simulink model "pathFollowingRobotPerturb"  (R2024b)
settings: Solver=VariableStepAuto  StartTime=0.0  StopTime=10000  RelTol=1e-3
undefined symbols (not defined in the file): a, angles, du, dw, dx, dy, initPose, leftPerturbT, mapMaxDimension, maxAngSpeed, maxLinSpeed, minAngSpeed, minLinSpeed, pathpoints, q1, q2, q3, q4, q5, q6, rightPerturbT, sampleTime, speeds
libraries: rllib x1
settings Model: SimulationMode=accelerator  SnapshotBufferSize=100  SnapshotInterval=100  PacingRate=1000  Creator=jose6  LastModifiedBy=jose6
settings DataIOCC: InspectSignalLogs=on

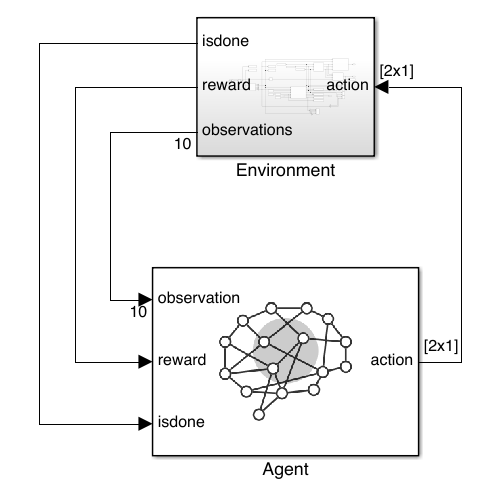
[thumbnail: Simulink's stored preview of the top-level diagram]
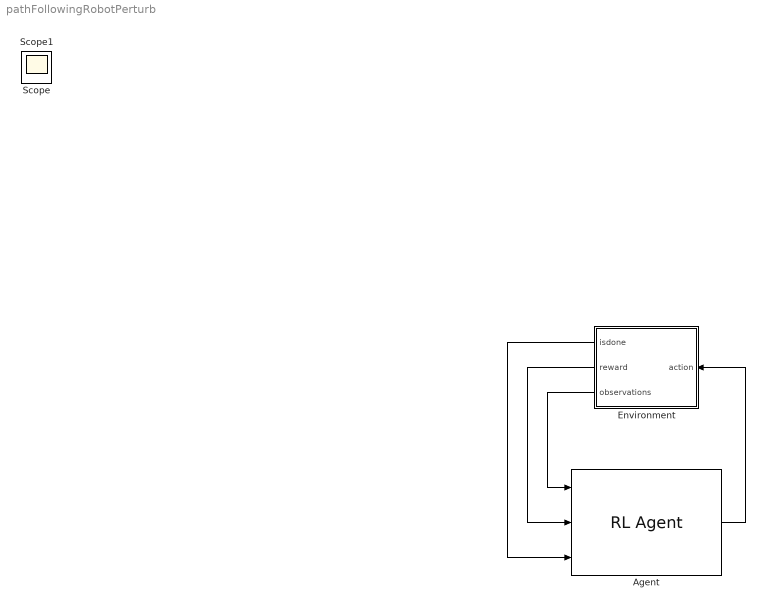
== system pathFollowingRobotPerturb ==
  Agent : rllib/RL Agent  Agent=agent  ExternalActionAsInput=off  ProvideLastAction=off  ProvideCumRwd=off  TreatAsDirectFeedthrough=on  UseStrictObservationDataTypes=off
  Environment : Subsystem
  Scope : Scope
  Scope1 : Scope
  wires:
  Agent/1 -> Environment/1(action)
  Environment/1(isdone) -> Agent/3
  Environment/2(reward) -> Agent/2
  Environment/3(observations) -> Agent/1

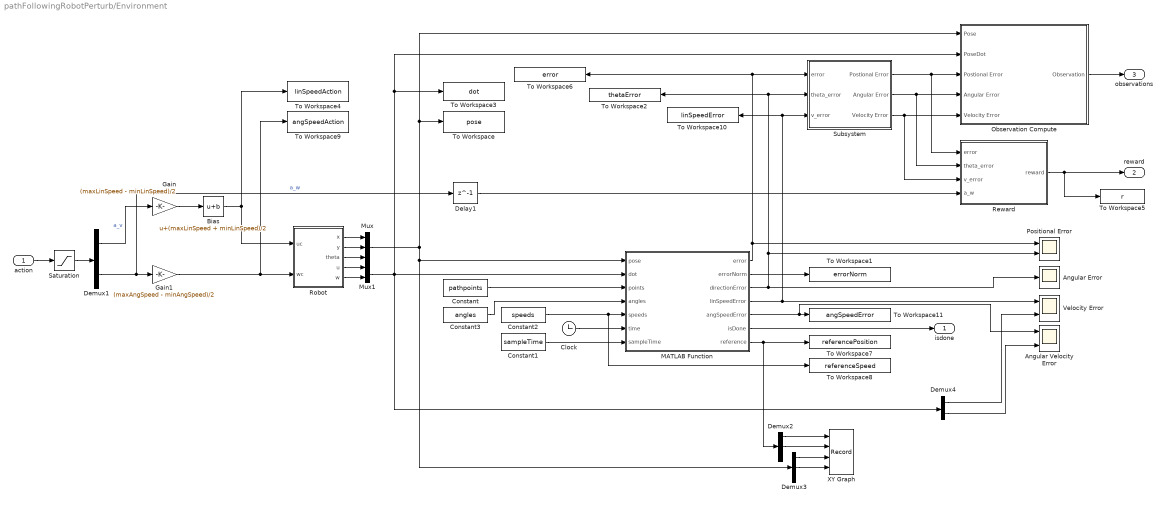
== system pathFollowingRobotPerturb/Environment ==
  action : Inport
  Angular Error : Scope
  Angular Velocity Error : Scope  NumInputPorts=2
  Bias : Bias  Bias=(maxLinSpeed + minLinSpeed)/2  SaturateOnIntegerOverflow=off
  Clock : Clock
  Constant : Constant  Value=pathpoints
  Constant1 : Constant  Value=sampleTime
  Constant2 : Constant  Value=speeds
  Constant3 : Constant  Value=angles
  Delay1 : Delay  DelayLength=1  InitialCondition=0  UseCircularBuffer=on
  Demux1 : Demux  Outputs=2
  Demux2 : Demux  Outputs=3
  Demux3 : Demux  Outputs=3
  Demux4 : Demux  Outputs=2
  Gain : Gain  Gain=(maxLinSpeed - minLinSpeed)/2
  Gain1 : Gain  Gain=(maxAngSpeed - minAngSpeed)/2
  MATLAB Function : MATLAB Function  TreatAsAtomicUnit=on
  Mux : Mux  Inputs=3
  Mux1 : Mux  Inputs=2
  Observation Compute : Subsystem
  Positional Error : Scope  NumInputPorts=2
  Reward : Subsystem
  Robot : Subsystem
  Saturation : Saturate  UpperLimit=1  LowerLimit=-1
  Subsystem : Subsystem
  To Workspace : ToWorkspace  VariableName=pose  SampleTime=-1
      settings: Save2DSignal=2-D array (concatenate along first dimension)
  To Workspace1 : ToWorkspace  VariableName=errorNorm  SampleTime=-1
      settings: Save2DSignal=2-D array (concatenate along first dimension)
  To Workspace10 : ToWorkspace  VariableName=linSpeedError  SampleTime=-1
      settings: Save2DSignal=2-D array (concatenate along first dimension)
  To Workspace11 : ToWorkspace  VariableName=angSpeedError  SampleTime=-1
      settings: Save2DSignal=2-D array (concatenate along first dimension)
  To Workspace2 : ToWorkspace  VariableName=thetaError  SampleTime=-1
      settings: Save2DSignal=2-D array (concatenate along first dimension)
  To Workspace3 : ToWorkspace  VariableName=dot  SampleTime=-1
      settings: Save2DSignal=2-D array (concatenate along first dimension)
  To Workspace4 : ToWorkspace  VariableName=linSpeedAction  SampleTime=-1
      settings: Save2DSignal=2-D array (concatenate along first dimension)
  To Workspace5 : ToWorkspace  VariableName=r  SampleTime=-1
      settings: Save2DSignal=2-D array (concatenate along first dimension)
  To Workspace6 : ToWorkspace  VariableName=error  SampleTime=-1
      settings: Save2DSignal=2-D array (concatenate along first dimension)
  To Workspace7 : ToWorkspace  VariableName=referencePosition  SampleTime=-1
      settings: Save2DSignal=2-D array (concatenate along first dimension)
  To Workspace8 : ToWorkspace  VariableName=referenceSpeed  SampleTime=-1
      settings: Save2DSignal=2-D array (concatenate along first dimension)
  To Workspace9 : ToWorkspace  VariableName=angSpeedAction  SampleTime=-1
      settings: Save2DSignal=2-D array (concatenate along first dimension)
  Velocity Error : Scope  NumInputPorts=2
  XY Graph : Record  FileSettingsInternal="{\"entries\":[{\"content\":{\"excelSettings\":{\"content\":{},\"type\":\"Streamout.ExcelSettings\"}},\"type\":\"Streamout.FileSettingStorage\",\"uuid\":\"\"}],\"packageUris\":[\"http:\\/\\/schema.mathworks.com\\/mf0\\/streamout_blocks\\/R2020a\"],\"version\":\"1.0\"}"  Layout=[1 1]  SignalsInternal="{\"entries\":[{\"content\":{\"signals\":[{\"content\":{\"blockPath\":[],\"dimensions\":[1],\"domain\":\"\",\"lineColor\":\"#d95319\",\"lineWidth\":2,\"plots\":[ 1 ],\"port\":1,\"sid\":[\"\"],\"signalID\":1,\"signalName\":\"Demux2:1\"},\"type\":\"RecordBlkView.Signal\",\"uuid\":\"\"},{\"content\":{\"blockPath\":[],\"dimensions\":[1],\"domain\":\"\",\"lineColor\":\"#22b573\",\"lineWidth\":2,\"plots\":[ 1 ],\"port\":2,\"sid\":[\"\"],\"signalID\":2,\"signalName\":\"Demux2:2\"},\"type\":\"RecordBlkView.Signal\",\"uuid\":\"\"},{\"content\":{\"blockPath\":[],\"dimensions\":[1],\"domain\":\"\",\"lineColor\":\"#0072bd\",\"lineWidth\":2,\"plots\":[ 1 ],\"port\":3,\"sid\":[\"\"],\"signalID\":3,\"signalName\":\"Demux3:1\"},\"type\":\"RecordBlkView.Signal\",\"uuid\":\"\"},{\"content\":{\"blockPath\":[],\"dimensions\":[1],\"domain\":\"\",\"lineColor\":\"#d95319\",\"lineWidth\":2,\"plots\":[ 1 ],\"port\":4,\"sid\":[\"\"],\"signalID\":4,\"signalName\":\"Demux3:2\"},\"type\":\"RecordBlkView.Signal\",\"uuid\":\"\"}]},\"type\":\"RecordBlkView.InputSignals\",\"uuid\":\"\"}],\"packageUris\":[\"http:\\/\\/schema.mathworks.com\\/mf0\\/streamout_blocks\\/R2020a\"],\"version\":\"1.0\"}"  VisualizationBindings="{\"xyplotplugin\":{\"info\":[{\"series\":[{\"bindingParametersList\":[{\"parameter\":\"X-Axis\",\"signalID\":3,\"signalName\":\"Demux3:1\"},{\"parameter\":\"Y-Axis\",\"signalID\":4,\"signalName\":\"Demux3:2\"},{\"parameter\":\"X-Axis\",\"signalID\":3,\"signalName\":\"Demux3:1\"},{\"parameter\":\"Y-Axis\",\"signalID\":4,\"signalName\":\"Demux3:2\"}],\"seriesID\":0},{\"bindingParametersList\":[{\"parameter\":\"X-Axis\",\"signalID\":1,\"signalName\":\"Demux2:1\"},{\"parameter\":\"Y-Axis\",\"signalID\":2,\"signalName\":\"Demux2:2\"}],\"seriesID\":1}],\"subplotID\":1}]}}"  CompatibilityTag=XY
  isdone : Outport
  reward : Outport  Port=2
  observations : Outport  Port=3
  wires:
  Constant/1 -> MATLAB Function/3(points)
  Gain/1 -> Bias/1
  action/1 -> Saturation/1
  Demux1/1 -> Gain/1  "a_v"
  Demux1/2 -> Delay1/1, Gain1/1  "a_w"
  Gain1/1 -> To Workspace9/1, Robot/2(wc)
  Reward/1(reward) -> To Workspace5/1, reward/1
  MATLAB Function/6(isDone) -> isdone/1
  Clock/1 -> MATLAB Function/6(time)
  Constant1/1 -> MATLAB Function/7(sampleTime)
  MATLAB Function/2(errorNorm) -> To Workspace1/1
  Observation Compute/1(Observation) -> observations/1
  Mux1/1 -> Demux4/1, Observation Compute/2(PoseDot), To Workspace3/1, MATLAB Function/2(dot)
  Bias/1 -> Robot/1(uc), To Workspace4/1
  Subsystem/1(Postional Error) -> Reward/1(error), Observation Compute/3(Postional Error)
  Subsystem/2(Angular Error) -> Reward/2(theta_error), Observation Compute/4(Angular Error)
  Robot/1(x) -> Mux/1
  Robot/3(theta) -> Mux/3
  Robot/5(w) -> Mux1/2
  Robot/2(y) -> Mux/2
  Robot/4(u) -> Mux1/1
  Saturation/1 -> Demux1/1
  Constant3/1 -> MATLAB Function/4(angles)
  Subsystem/3(Velocity Error) -> Reward/3(v_error), Observation Compute/5(Velocity Error)
  Delay1/1 -> Reward/4(a_w)
  MATLAB Function/1(error) -> Subsystem/1(error), To Workspace6/1, Positional Error/1
  MATLAB Function/3(directionError) -> Subsystem/2(theta_error), To Workspace2/1, Positional Error/2, Angular Error/1
  Constant2/1 -> To Workspace8/1, MATLAB Function/5(speeds)
  MATLAB Function/4(linSpeedError) -> Subsystem/3(v_error), To Workspace10/1, Velocity Error/1
  MATLAB Function/5(angSpeedError) -> Angular Velocity Error/1, To Workspace11/1
  Demux4/1 -> Velocity Error/2
  Demux4/2 -> Angular Velocity Error/2
  Mux/1 -> Demux3/1, MATLAB Function/1(pose), Observation Compute/1(Pose), To Workspace/1
  MATLAB Function/7(reference) -> To Workspace7/1, Demux2/1
  Demux3/1 -> XY Graph/3
  Demux3/2 -> XY Graph/4
  Demux2/1 -> XY Graph/1
  Demux2/2 -> XY Graph/2

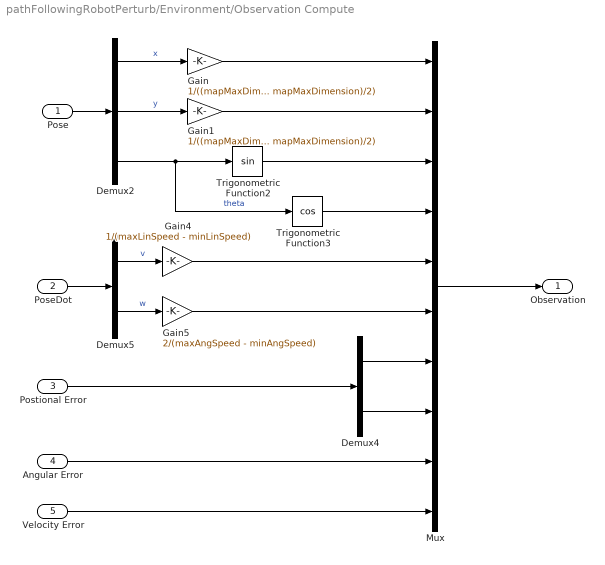
== system pathFollowingRobotPerturb/Environment/Observation Compute ==
  Pose : Inport
  PoseDot : Inport  Port=2
  Postional Error : Inport  Port=3
  Angular Error : Inport  Port=4
  Velocity Error : Inport  Port=5
  Demux2 : Demux  Outputs=3
  Demux4 : Demux  Outputs=2
  Demux5 : Demux  Outputs=2
  Gain : Gain  Gain=1/((mapMaxDimension + mapMaxDimension)/2)
  Gain1 : Gain  Gain=1/((mapMaxDimension + mapMaxDimension)/2)
  Gain4 : Gain  Gain=1/(maxLinSpeed - minLinSpeed)
  Gain5 : Gain  Gain=2/(maxAngSpeed - minAngSpeed)
  Mux : Mux  Inputs=10
  Trigonometric Function2 : Trigonometry
  Trigonometric Function3 : Trigonometry  Operator=cos
  Observation : Outport
  wires:
  Demux4/2 -> Mux/8
  Demux2/2 -> Gain1/1  "y"
  Demux4/1 -> Mux/7
  Postional Error/1 -> Demux4/1
  Mux/1 -> Observation/1
  Pose/1 -> Demux2/1
  Demux2/1 -> Gain/1  "x"
  Velocity Error/1 -> Mux/10
  Gain/1 -> Mux/1
  Gain1/1 -> Mux/2
  Angular Error/1 -> Mux/9
  Demux2/3 -> Trigonometric Function2/1, Trigonometric Function3/1  "theta"
  Trigonometric Function3/1 -> Mux/4
  Trigonometric Function2/1 -> Mux/3
  PoseDot/1 -> Demux5/1
  Gain4/1 -> Mux/5
  Gain5/1 -> Mux/6
  Demux5/1 -> Gain4/1  "v"
  Demux5/2 -> Gain5/1  "w"

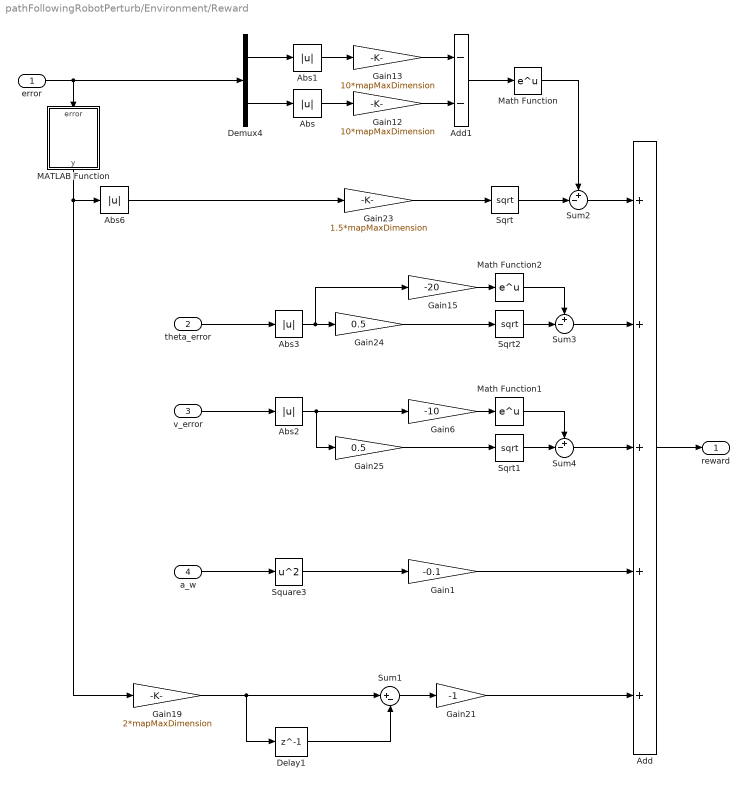
== system pathFollowingRobotPerturb/Environment/Reward ==
  error : Inport
  theta_error : Inport  Port=2
  v_error : Inport  Port=3
  a_w : Inport  Port=4
  Abs{,1..3,6} (5 alike) : Abs  SaturateOnIntegerOverflow=off
  Add : Sum  Inputs=+++++
  Add1 : Sum  Inputs=--
  Delay1 : Delay  DelayLength=1  InitialCondition=0  UseCircularBuffer=on
  Demux4 : Demux  Outputs=2
  Gain1 : Gain  Gain=-0.1
  Gain12 : Gain  Gain=10*mapMaxDimension
  Gain13 : Gain  Gain=10*mapMaxDimension
  Gain15 : Gain  Gain=-20
  Gain19 : Gain  Gain=2*mapMaxDimension
  Gain21 : Gain  Gain=-1
  Gain23 : Gain  Gain=1.5*mapMaxDimension
  Gain24 : Gain  Gain=0.5
  Gain25 : Gain  Gain=0.5
  Gain6 : Gain  Gain=-10
  MATLAB Function : MATLAB Function  TreatAsAtomicUnit=on
  Math Function : Math
  Math Function1 : Math
  Math Function2 : Math
  Sqrt : Sqrt
  Sqrt1 : Sqrt
  Sqrt2 : Sqrt
  Square3 : Math  Operator=square  SignedPower=on  RndMeth=Zero
  Sum1 : Sum  Inputs=|+-
  Sum2 : Sum  Inputs=+-|
  Sum3 : Sum  Inputs=+-|
  Sum4 : Sum  Inputs=+-|
  reward : Outport
  wires:
  Square3/1 -> Gain1/1
  Add1/1 -> Math Function/1
  Abs3/1 -> Gain15/1, Gain24/1
  Abs2/1 -> Gain25/1, Gain6/1
  Gain13/1 -> Add1/1
  Gain12/1 -> Add1/2
  Gain19/1 -> Sum1/1, Delay1/1
  Sum1/1 -> Gain21/1
  Delay1/1 -> Sum1/2
  theta_error/1 -> Abs3/1
  v_error/1 -> Abs2/1
  error/1 -> MATLAB Function/1(error), Demux4/1
  Add/1 -> reward/1
  a_w/1 -> Square3/1
  MATLAB Function/1(y) -> Gain19/1, Abs6/1
  Gain15/1 -> Math Function2/1
  Gain6/1 -> Math Function1/1
  Demux4/1 -> Abs1/1
  Demux4/2 -> Abs/1
  Abs/1 -> Gain12/1
  Abs1/1 -> Gain13/1
  Sqrt/1 -> Sum2/2
  Sqrt2/1 -> Sum3/2
  Sqrt1/1 -> Sum4/2
  Gain24/1 -> Sqrt2/1
  Gain25/1 -> Sqrt1/1
  Gain21/1 -> Add/5
  Math Function1/1 -> Sum4/1
  Math Function2/1 -> Sum3/1
  Sum2/1 -> Add/1
  Math Function/1 -> Sum2/1
  Gain23/1 -> Sqrt/1
  Abs6/1 -> Gain23/1
  Sum3/1 -> Add/2
  Gain1/1 -> Add/4
  Sum4/1 -> Add/3

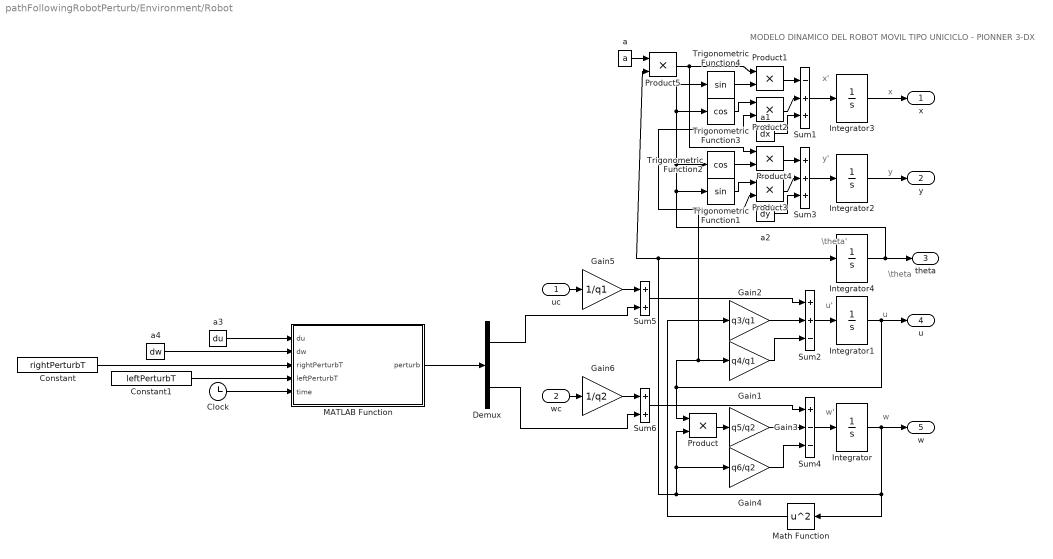
== system pathFollowingRobotPerturb/Environment/Robot ==
  note: u'
  note: u
  note: x'
  note: x
  note: y'
  note: y
  note: \theta
  note: w
  note: w'
  note: \theta'
  note: MODELO DINAMICO DEL ROBOT MOVIL TIPO UNICICLO - PIONNER 3-DX
  uc : Inport
  wc : Inport  Port=2
  Clock : Clock
  Constant : Constant  Value=rightPerturbT
  Constant1 : Constant  Value=leftPerturbT
  Demux : Demux  Outputs=2
  Gain1 : Gain  Gain=q4/q1  SaturateOnIntegerOverflow=on  OutDataTypeStr=Inherit: Same as input  ParamDataTypeStr=Inherit: Same as input
  Gain2 : Gain  Gain=q3/q1  SaturateOnIntegerOverflow=on  OutDataTypeStr=Inherit: Same as input  ParamDataTypeStr=Inherit: Same as input
  Gain3 : Gain  Gain=q5/q2  SaturateOnIntegerOverflow=on  OutDataTypeStr=Inherit: Same as input  ParamDataTypeStr=Inherit: Same as input
  Gain4 : Gain  Gain=q6/q2  SaturateOnIntegerOverflow=on  OutDataTypeStr=Inherit: Same as input  ParamDataTypeStr=Inherit: Same as input
  Gain5 : Gain  Gain=1/q1  SaturateOnIntegerOverflow=on  OutDataTypeStr=Inherit: Same as input  ParamDataTypeStr=Inherit: Same as input
  Gain6 : Gain  Gain=1/q2  SaturateOnIntegerOverflow=on  OutDataTypeStr=Inherit: Same as input  ParamDataTypeStr=Inherit: Same as input
  Integrator : Integrator
  Integrator1 : Integrator
  Integrator2 : Integrator  InitialCondition=initPose(2)
  Integrator3 : Integrator  InitialCondition=initPose(1)
  Integrator4 : Integrator  InitialCondition=initPose(3)
  MATLAB Function : MATLAB Function  TreatAsAtomicUnit=on
  Math Function : Math  Operator=square  SignedPower=on
  Product{,1..5} (6 alike) : Product  SaturateOnIntegerOverflow=on  OutDataTypeStr=Inherit: Same as first input
  Sum1 : Sum  Inputs=-++  InputSameDT=on  SaturateOnIntegerOverflow=on  OutDataTypeStr=Inherit: Same as first input
  Sum2 : Sum  Inputs=++-  InputSameDT=on  SaturateOnIntegerOverflow=on  OutDataTypeStr=Inherit: Same as first input
  Sum3 : Sum  Inputs=+++  InputSameDT=on  SaturateOnIntegerOverflow=on  OutDataTypeStr=Inherit: Same as first input
  Sum4 : Sum  Inputs=+--  InputSameDT=on  SaturateOnIntegerOverflow=on  OutDataTypeStr=Inherit: Same as first input
  Sum5 : Sum  InputSameDT=on  SaturateOnIntegerOverflow=on  OutDataTypeStr=Inherit: Same as first input
  Sum6 : Sum  InputSameDT=on  SaturateOnIntegerOverflow=on  OutDataTypeStr=Inherit: Same as first input
  Trigonometric Function1 : Trigonometry
  Trigonometric Function2 : Trigonometry  Operator=cos
  Trigonometric Function3 : Trigonometry  Operator=cos
  Trigonometric Function4 : Trigonometry
  a : Constant  Value=a
  a1 : Constant  Value=dx
  a2 : Constant  Value=dy
  a3 : Constant  Value=du
  a4 : Constant  Value=dw
  x : Outport  InitialOutput=0
  y : Outport  Port=2  InitialOutput=0
  theta : Outport  Port=3  InitialOutput=0
  u : Outport  Port=4  InitialOutput=0
  w : Outport  Port=5  InitialOutput=0
  wires:
  Sum2/1 -> Integrator1/1
  Integrator1/1 -> u/1, Product/1, Gain1/1, Product3/2, Product2/2
  Sum1/1 -> Integrator3/1
  Integrator3/1 -> x/1
  Product1/1 -> Sum1/1
  Sum3/1 -> Integrator2/1
  Integrator2/1 -> y/1
  Product4/1 -> Sum3/1
  Integrator4/1 -> theta/1, Trigonometric Function2/1, Trigonometric Function4/1, Trigonometric Function3/1, Trigonometric Function1/1
  Trigonometric Function2/1 -> Product4/2
  Trigonometric Function4/1 -> Product1/2
  Product3/1 -> Sum3/2
  Product2/1 -> Sum1/2
  Trigonometric Function3/1 -> Product2/1
  Trigonometric Function1/1 -> Product3/1
  Integrator/1 -> w/1, Math Function/1, Gain4/1, Product/2, Product5/2, Integrator4/1
  Sum4/1 -> Integrator/1
  Gain2/1 -> Sum2/2
  Math Function/1 -> Gain2/1
  Gain1/1 -> Sum2/3
  Gain3/1 -> Sum4/2
  Gain4/1 -> Sum4/3
  Product/1 -> Gain3/1
  uc/1 -> Gain5/1
  wc/1 -> Gain6/1
  Sum5/1 -> Sum2/1
  Sum6/1 -> Sum4/1
  Gain5/1 -> Sum5/1
  Gain6/1 -> Sum6/1
  a1/1 -> Sum1/3
  a2/1 -> Sum3/3
  a/1 -> Product5/1
  Product5/1 -> Product1/1, Product4/1
  Constant/1 -> MATLAB Function/3(rightPerturbT)
  Demux/1 -> Sum5/2
  Demux/2 -> Sum6/2
  Constant1/1 -> MATLAB Function/4(leftPerturbT)
  MATLAB Function/1(perturb) -> Demux/1
  Clock/1 -> MATLAB Function/5(time)
  a3/1 -> MATLAB Function/1(du)
  a4/1 -> MATLAB Function/2(dw)

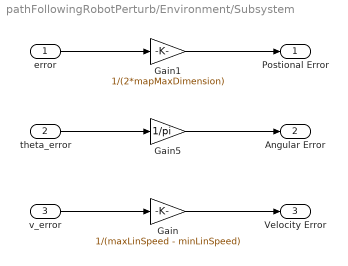
== system pathFollowingRobotPerturb/Environment/Subsystem ==
  error : Inport
  theta_error : Inport  Port=2
  v_error : Inport  Port=3
  Gain : Gain  Gain=1/(maxLinSpeed - minLinSpeed)
  Gain1 : Gain  Gain=1/(2*mapMaxDimension)
  Gain5 : Gain  Gain=1/pi
  Postional Error : Outport
  Angular Error : Outport  Port=2
  Velocity Error : Outport  Port=3
  wires:
  theta_error/1 -> Gain5/1
  Gain5/1 -> Angular Error/1
  error/1 -> Gain1/1
  Gain1/1 -> Postional Error/1
  v_error/1 -> Gain/1
  Gain/1 -> Velocity Error/1

== matlab function pathFollowingRobotPerturb/Environment/MATLAB Function ==
  settings: updateMethod=DISCRETE
  data: pose input size=3; dot input; points input; angles input; speeds input; time input; error output; errorNorm output; directionError output; linSpeedError output; angSpeedError output; isDone output; sampleTime input; reference output
function [error, errorNorm, directionError, linSpeedError, angSpeedError, isDone, reference] = progress(pose, dot, points, angles, speeds, time, sampleTime) %#codegen
[error, errorNorm, directionError, linSpeedError, angSpeedError, isDone, reference, nextReference] = support.computeProgress(pose, dot, speeds, time, points, angles, sampleTime);

== matlab function pathFollowingRobotPerturb/Environment/Reward/MATLAB Function ==
  data: error input; y output
function y = error_norm(error)

y = norm(error);

== matlab function pathFollowingRobotPerturb/Environment/Robot/MATLAB Function ==
  data: du input; dw input; rightPerturbT input; perturb output; leftPerturbT input; time input
function perturb = fcn(du, dw, rightPerturbT, leftPerturbT, time)
if round(time) == round(rightPerturbT)
    perturb = [du dw];
elseif round(time) == round(leftPerturbT)
    perturb = [-du -dw];
else
    perturb = [0 0];
end
end
